simulink model "power_FlybackConverter"  (R2022a)
settings: Solver=VariableStepAuto  StartTime=0.0  StopTime=0.1  MaxStep=1e-4  RelTol=1e-4  EnableMultiTasking=on
libraries: spsSeriesRLCBranchLib x2, spsDiodeLib x2, spsMultimeterLib x2, spsLinearTransformerLib x1, spsMosfetLib x1, spsMeanLib x1, spsParallelRLCBranchLib x1, spsDCVoltageSourceLib x1, spsVoltageMeasurementLib x1, spspowerguiLib x1
settings Model: Creator=The MathWorks, Inc.  LastModifiedBy=kkaya674
settings SolverCC: AlgebraicLoopSolver=TrustRegion  SolverResetMethod=Robust
settings OptimizationCC: LifeSpan=inf
settings DebuggingCC: ReadBeforeWriteMsg=DisableAll  WriteAfterWriteMsg=DisableAll  WriteAfterReadMsg=DisableAll  MultiTaskDSMMsg=none  UnconnectedInputMsg=warning  UnconnectedOutputMsg=warning  UnconnectedLineMsg=warning  SFUnexpectedBacktrackingDiag=warning  SFNoUnconditionalDefaultTransitionDiag=warning  SFExecutionAtInitializationDiag=none  SFMachineParentedDataDiag=warning  ArithmeticOperatorsInVariantConditions=warning
settings ModelReferenceCC: UpdateModelReferenceTargets=IfOutOfDate
settings SFSimCC: SFSimEcho=off  SimUseLocalCustomCode=off  CustomCodeUndefinedFunction=UseInterfaceOnly
settings RTWCC: RTWUseLocalCustomCode=off
settings CodeAppCC: StateflowObjectComments=on
settings GRTTargetCC: TargetLangStandard=C89/C90 (ANSI)
settings ConfigComp: CovMetricSettings=dw  CovSaveCumulativeToWorkspaceVar=on  CovSaveSingleToWorkspaceVar=on  CovExternalEMLEnable=off
settings SimscapeCC: SimscapeNormalizeSystem=off  SimscapeNominalValues={1, 'bar'; 1, 'cm^3/s'; 1, 'bar*kg/s'; 1, 'kJ/kg'; 1, 'kW'; }

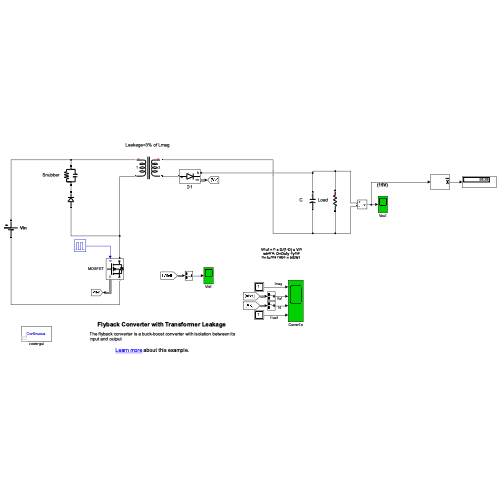
[thumbnail: Simulink's stored preview of the top-level diagram]
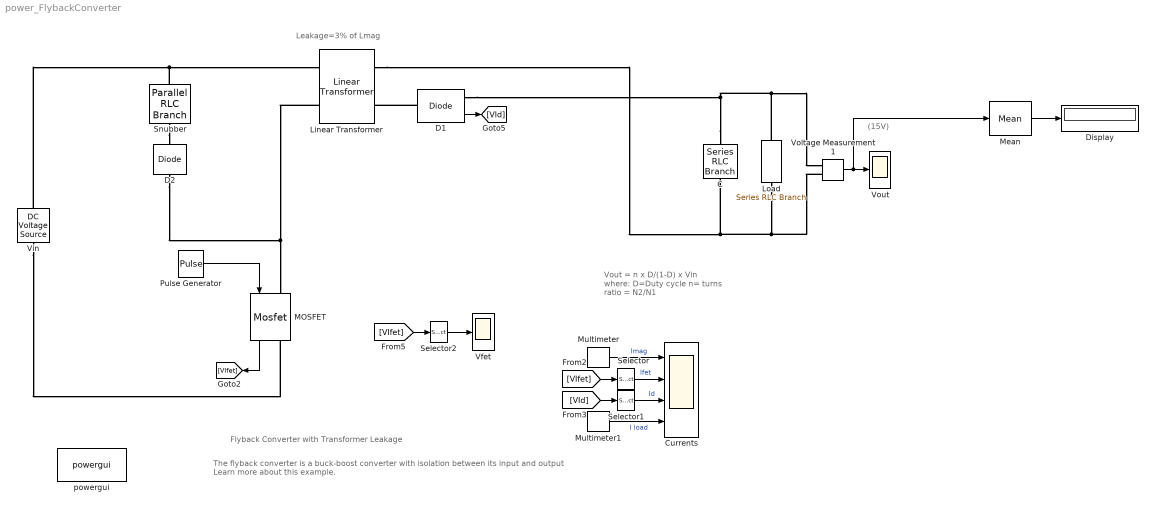
== system power_FlybackConverter ==
  note: (15V)
  note: Leakage=3% of Lmag
  note: Vout = n x D/(1-D) x Vin
      | where: D=Duty cycle
      | n= turns ratio = N2/N1
  note: Flyback Converter with Transformer Leakage
  note: The flyback converter is a buck-boost converter with isolation between its input and output
      |
      | Learn more about this example.
  C : spsSeriesRLCBranchLib/Series RLC Branch  LConnTagsString=__new0  RConnTagsString=__new0  BranchType=C  Resistance=1e-4  Inductance=200e-6  SetiL0=off  InitialCurrent=0  Capacitance=200e-6  Setx0=off  InitialVoltage=0  Measurements=None
  Currents : Scope  NumInputPorts=4
  D1 : spsDiodeLib/Diode  Ron=1e-3  Lon=0  Vf=0  IC=0  UseSnubber=off  Rs=inf  Cs=0  Measurements=on
  D2 : spsDiodeLib/Diode  Ron=1e-3  Lon=0  Vf=0  IC=0  UseSnubber=off  Rs=inf  Cs=0  Measurements=off
  Display : Display
  Linear Transformer : spsLinearTransformerLib/Linear Transformer  UNITS=SI  NominalPower=[ 10e5 100e3 ]  winding1=[30 0 3e-6]  winding2=[30 0 0]  ThreeWindings=off  winding3=[3.15e+05 3.969e+07 6316.9]  RmLm=[1e4 1000e-6]  Measurements=Magnetization current  DataType=on
  Load : spsSeriesRLCBranchLib/Series RLC Branch  LConnTagsString=__new0  RConnTagsString=__new0  BranchType=R  Resistance=5  Inductance=200e-6  SetiL0=off  InitialCurrent=0  Capacitance=400e-6  Setx0=off  InitialVoltage=0  Measurements=Branch current
  MOSFET : spsMosfetLib/Mosfet  Ron=1e-3  Lon=0  Rd=1e-3  Vfd=0  IC=0  Rs=1e6  Cs=inf  Measurements=on
  Mean : spsMeanLib/Mean  Freq=100000  Vinit=0  Ts=0
  Multimeter : spsMultimeterLib/Multimeter  L=4  sel=4  yselected={}  Gain=1  OutputType=Complex  PlotAtSimulationStop=off  PhasorSimulation=off
  Multimeter1 : spsMultimeterLib/Multimeter  L=4  sel=1  yselected={}  Gain=1  OutputType=Complex  PlotAtSimulationStop=off  PhasorSimulation=off
  Pulse Generator : DiscretePulseGenerator  PulseType=Time based  Period=1/10e3  PulseWidth=66
  Selector : Selector  InputPortWidth=2  IndexOptions=Index vector (dialog)  Indices=1  OutputSizes=1
  Selector1 : Selector  InputPortWidth=2  IndexOptions=Index vector (dialog)  Indices=1  OutputSizes=1
  Selector2 : Selector  InputPortWidth=2  IndexOptions=Index vector (dialog)  Indices=2  OutputSizes=1
  Snubber : spsParallelRLCBranchLib/Parallel RLC Branch  LConnTagsString=a  RConnTagsString=__new0  BranchType=RC  Resistance=10e3  Inductance=1e-3  SetiL0=off  InitialCurrent=0  Capacitance=47e-9  Setx0=off  InitialVoltage=0  Measurements=None
  Vfet : Scope
  Vin : spsDCVoltageSourceLib/DC Voltage Source  Amplitude=30  Measurements=None
  Voltage Measurement1 : spsVoltageMeasurementLib/Voltage Measurement  PhasorSimulation=off  OutputType=Complex  PSBequivalent=0
  Vout : Scope
  powergui : spspowerguiLib/powergui  Priority=1  SimulationMode=Continuous  SampleTime=50e-6  frequency=60  Iterations=50  frequencyindice=0  Pbase=100e6  ErrMax=1e-4  UnitsV=kV  UnitsW=MW  buscounter=0  FunctionMessages=off  echomessages=off  EnableUseOfTLC=off  CurrentSourceSwitches=off  DisableSnubberDevices=off  DisableRonSwitches=off  DisableVfSwitches=off  DisplayEquations=off  AutomaticDiscreteSolvers=off  SolverType=Tustin/Backward Euler (TBE)  Interpol=off  ExternalGateDelay=off  methode=off  Ts=100  x0status=blocks  SPID=on  SwTol=0  HookPort=off  NonlinearTolerance=1e-4  nMaxIteration=100  ContinueOnMaxIteration=off  RestoreLinks=warning  ResistiveCurrentMeasurement=off  Frange=[0:2:500]  Ylog=off  Xlog=on  ShowGrid=off  save=off  variable=ZData  structure=0  ZoomFFT=off  StartTime=0.0  cycles=1  DisplayStyle=1  fundamental=60  FreqAxis=off  MaxFrequency=1000  frequencyindicesteady=1  RmsSteady=1  display=off
  wires:
  Pulse Generator/1 -> MOSFET/1
  Voltage Measurement1/1 -> Mean/1, Vout/1
  MOSFET/1 -> [VIfet]
  D1/1 -> [VId]
  Multimeter/1 -> Currents/1  "Imag"
  Selector/1 -> Currents/2  "Ifet"
  [VIfet] -> Selector/1
  Selector1/1 -> Currents/3  "Id"
  [VId] -> Selector1/1
  Multimeter1/1 -> Currents/4  "I load"
  Selector2/1 -> Vfet/1
  [VIfet] -> Selector2/1
  Mean/1 -> Display/1
  connections:
  C/LConn1 -- D1/RConn1 -- Voltage Measurement1/LConn1 -- Load/LConn1
  Load/RConn1 -- Voltage Measurement1/LConn2 -- Linear Transformer/RConn1 -- C/RConn1
  Linear Transformer/LConn2 -- D2/LConn1 -- MOSFET/LConn1
  D1/LConn1 -- Linear Transformer/RConn2
  Snubber/RConn1 -- D2/RConn1
  Vin/LConn1 -- MOSFET/RConn1
  Vin/RConn1 -- Linear Transformer/LConn1 -- Snubber/LConn1
